simulink model "Encoder4_2"  (R2025b)
settings: Solver=VariableStepAuto  StartTime=0.0  StopTime=10.0  RelTol=1e-3
settings Model: Creator=Johan  LastModifiedBy=Johan

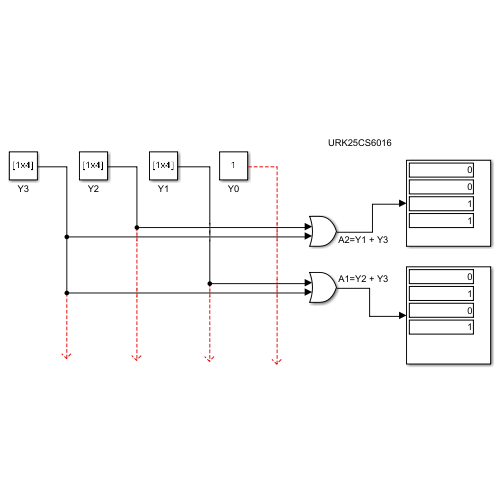
[thumbnail: Simulink's stored preview of the top-level diagram]
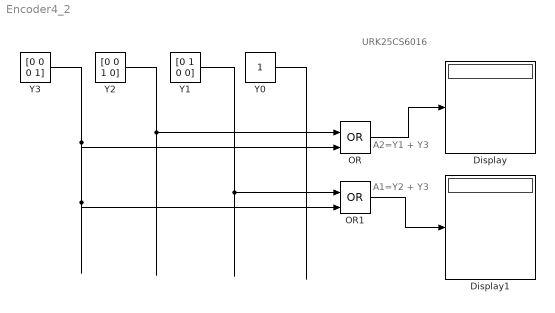
== system Encoder4_2 ==
  note: URK25CS6016
  note: A2=Y1 + Y3
  note: A1=Y2 + Y3
  Display : Display
  Display1 : Display
  OR : Logic  Operator=OR  IconShape=distinctive  AllPortsSameDT=off  OutDataTypeStr=boolean
  OR1 : Logic  Operator=OR  IconShape=distinctive  AllPortsSameDT=off  OutDataTypeStr=boolean
  Y0 : Constant
  Y1 : Constant  Value=[0 1 0 0]
  Y2 : Constant  Value=[0 0 1 0]
  Y3 : Constant  Value=[0 0 0 1]
  wires:
  Y0/1 -> ?
  Y1/1 -> OR1/1
  Y2/1 -> OR/1
  Y3/1 -> OR/2, OR1/2
  OR/1 -> Display/1
  OR1/1 -> Display1/1
